simulink model "model3"  (R2023a)
settings: Solver=VariableStepAuto  StartTime=0.0  StopTime=10.0  RelTol=1e-3
values from neighbouring files (symbols this model uses):
  A = [0, 1, 0, 0 ... (first row only)    [e01.m]
  B = [0, 0 ... (first row only)    [e01.m]
  C = [1, 0, 0, 0 ... (first row only)    [e01.m]
  D = [0, 0 ... (first row only)    [e01.m]
  L = L1'    [e01.m]
settings Model: Creator=Anirvan Krishna  LastModifiedBy=Anirvan Krishna

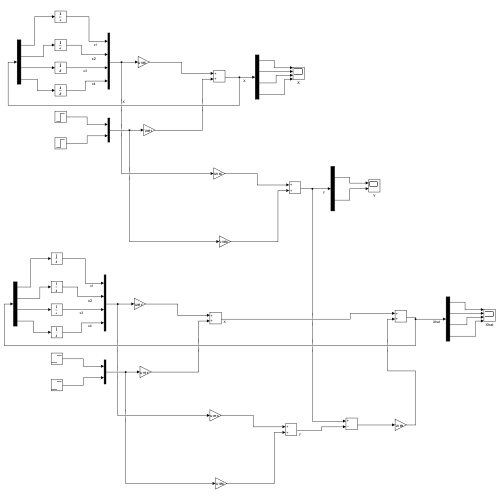
[thumbnail: Simulink's stored preview of the top-level diagram]
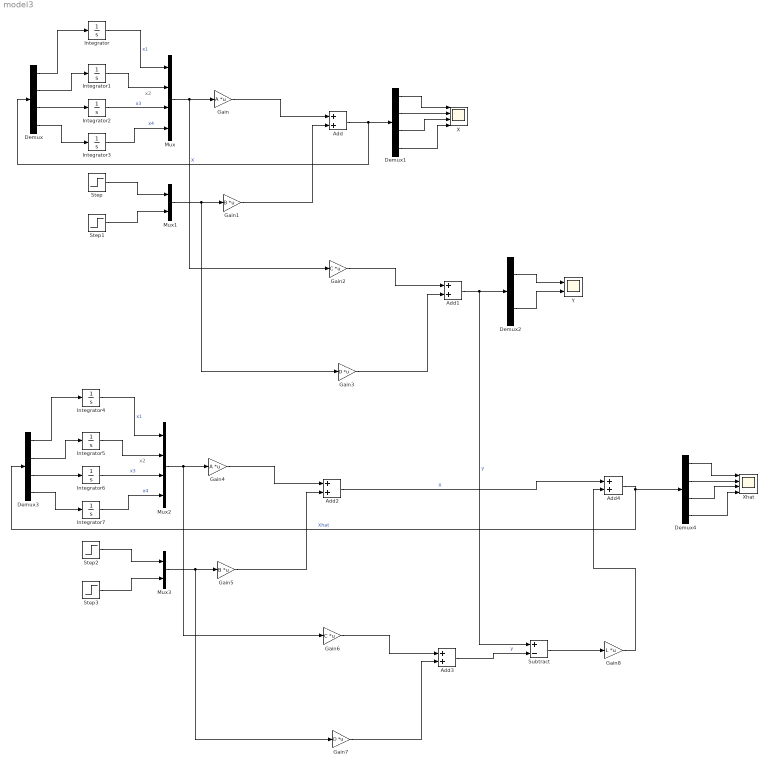
== system model3 ==
  note: x2
  note: x2
  Add{,1..4} (5 alike) : Sum
  Demux{,1,3..4} (4 alike) : Demux
  Demux2 : Demux  Outputs=2
  Gain : Gain  Gain=A  Multiplication=Matrix(K*u) (u vector)
  Gain1 : Gain  Gain=B  Multiplication=Matrix(K*u) (u vector)
  Gain2 : Gain  Gain=C  Multiplication=Matrix(K*u) (u vector)
  Gain3 : Gain  Gain=D  Multiplication=Matrix(K*u) (u vector)
  Gain4 : Gain  Gain=A  Multiplication=Matrix(K*u) (u vector)
  Gain5 : Gain  Gain=B  Multiplication=Matrix(K*u) (u vector)
  Gain6 : Gain  Gain=C  Multiplication=Matrix(K*u) (u vector)
  Gain7 : Gain  Gain=D  Multiplication=Matrix(K*u) (u vector)
  Gain8 : Gain  Gain=L  Multiplication=Matrix(K*u) (u vector)
  Integrator{,1..7} (8 alike) : Integrator
  Mux : Mux
  Mux1 : Mux  Inputs=2
  Mux2 : Mux
  Mux3 : Mux  Inputs=2
  Step{,1..3} (4 alike) : Step  Time=0  SampleTime=0
  Subtract : Sum  Inputs=+-
  X : Scope  NumInputPorts=4
  Xhat : Scope  NumInputPorts=4
  Y : Scope  NumInputPorts=2
  wires:
  Demux1/2 -> X/2
  Demux1/1 -> X/1
  Demux1/3 -> X/3
  Add1/1 -> Subtract/1, Demux2/1  "y"
  Demux2/1 -> Y/1
  Gain2/1 -> Add1/1
  Gain3/1 -> Add1/2
  Step1/1 -> Mux1/2
  Add/1 -> Demux1/1, Demux/1  "X"
  Demux2/2 -> Y/2
  Demux/3 -> Integrator2/1
  Demux/2 -> Integrator1/1
  Mux/1 -> Gain2/1, Gain/1
  Gain1/1 -> Add/2
  Step/1 -> Mux1/1
  Gain/1 -> Add/1
  Integrator2/1 -> Mux/3  "x3"
  Demux1/4 -> X/4
  Mux1/1 -> Gain3/1, Gain1/1
  Demux/4 -> Integrator3/1
  Demux/1 -> Integrator/1
  Integrator1/1 -> Mux/2
  Integrator3/1 -> Mux/4  "x4"
  Integrator/1 -> Mux/1  "x1"
  Gain4/1 -> Add2/1
  Demux3/1 -> Integrator4/1
  Gain5/1 -> Add2/2
  Mux2/1 -> Gain6/1, Gain4/1
  Step2/1 -> Mux3/1
  Integrator6/1 -> Mux2/3  "x3"
  Integrator7/1 -> Mux2/4  "x4"
  Integrator5/1 -> Mux2/2
  Gain7/1 -> Add3/2
  Step3/1 -> Mux3/2
  Mux3/1 -> Gain7/1, Gain5/1
  Demux3/2 -> Integrator5/1
  Demux3/3 -> Integrator6/1
  Demux3/4 -> Integrator7/1
  Gain6/1 -> Add3/1
  Integrator4/1 -> Mux2/1  "x1"
  Add3/1 -> Subtract/2  "y"
  Subtract/1 -> Gain8/1
  Gain8/1 -> Add4/2
  Add2/1 -> Add4/1  "X"
  Demux4/3 -> Xhat/3
  Add4/1 -> Demux4/1, Demux3/1  "Xhat"
  Demux4/4 -> Xhat/4
  Demux4/1 -> Xhat/1
  Demux4/2 -> Xhat/2
